simulink model "Ejer2P2"  (R2024b)
settings: Solver=VariableStepAuto  StartTime=0.0  StopTime=10.0  RelTol=1e-3
settings Model: Creator=lopez  LastModifiedBy=lopez

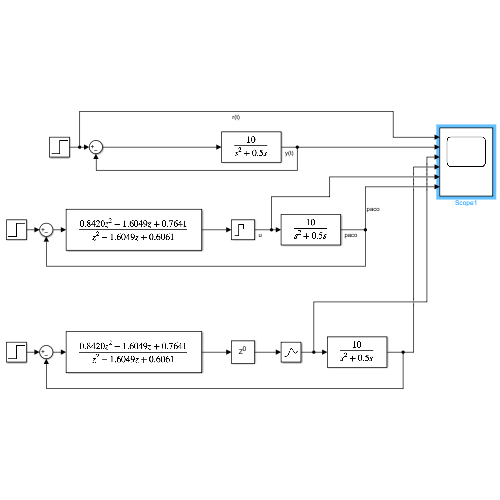
[thumbnail: Simulink's stored preview of the top-level diagram]
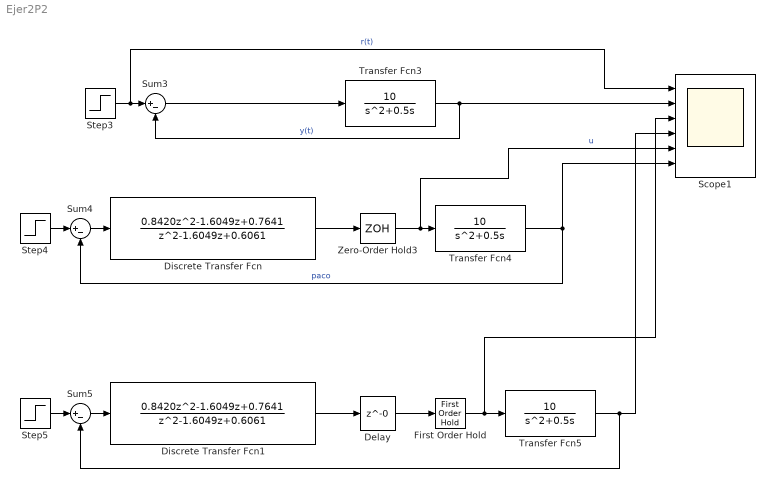
== system Ejer2P2 ==
  Delay : Delay  DelayLength=0  SampleTime=0.1
  Discrete Transfer Fcn : DiscreteTransferFcn  Numerator="[0.8420  -1.6049  0.7641]"  Denominator=[1 -1.6049 0.6061]
  Discrete Transfer Fcn1 : DiscreteTransferFcn  Numerator=[0.8420 -1.6049 0.7641]  Denominator=[1 -1.6049 0.6061]
  First Order Hold : FirstOrderHold  ErrorTolerance=inf
  Scope1 : Scope  NumInputPorts=6
  Step3 : Step  Time=0  Before=1  SampleTime=0
  Step4 : Step  Time=0  Before=1  SampleTime=0
  Step5 : Step  Time=0  Before=1  SampleTime=0
  Sum3 : Sum  Inputs=|+-
  Sum4 : Sum  Inputs=|+-
  Sum5 : Sum  Inputs=|+-
  Transfer Fcn3 : TransferFcn  Numerator=[10]  Denominator=[1 0.5 0]
  Transfer Fcn4 : TransferFcn  Numerator=[10]  Denominator=[1 0.5 0]
  Transfer Fcn5 : TransferFcn  Numerator=[10]  Denominator=[1 0.5 0]
  Zero-Order Hold3 : ZeroOrderHold  SampleTime=-1
  wires:
  Zero-Order Hold3/1 -> Scope1/5, Transfer Fcn4/1  "u"
  Step4/1 -> Sum4/1
  Sum5/1 -> Discrete Transfer Fcn1/1
  Sum4/1 -> Discrete Transfer Fcn/1
  First Order Hold/1 -> Scope1/3, Transfer Fcn5/1
  Sum3/1 -> Transfer Fcn3/1
  Step3/1 -> Scope1/1, Sum3/1  "r(t)"
  Delay/1 -> First Order Hold/1
  Transfer Fcn4/1 -> Scope1/6, Sum4/2  "paco"
  Discrete Transfer Fcn/1 -> Zero-Order Hold3/1
  Discrete Transfer Fcn1/1 -> Delay/1
  Step5/1 -> Sum5/1
  Transfer Fcn3/1 -> Sum3/2, Scope1/2  "y(t)"
  Transfer Fcn5/1 -> Sum5/2, Scope1/4
